simulink model "DC_gen_DC_PES"  (R2025a)
settings: Solver=VariableStepAuto  StartTime=0.0  StopTime=10.0  RelTol=1e-3
undefined symbols (not defined in the file): Grid_DCop_DC_PES
settings Model: Creator=atomas  LastModifiedBy=atomas

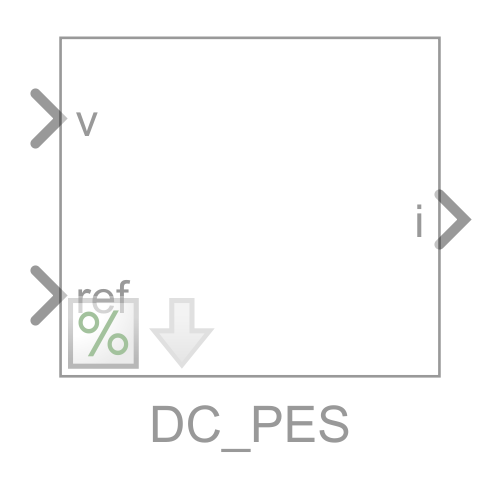
[thumbnail: Simulink's stored preview of the top-level diagram]
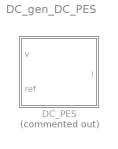
== system DC_gen_DC_PES ==
  DC_PES : Subsystem  Commented=on
      mask init:
      | mdlWks = get_param(bdroot,'ModelWorkspace'); % Get the model workspace
      | block_name = get_param(gcb,'Name');
      | try
      |     bvarname = get_param(get_param(get_param(...
      |         gcb, 'Parent'), 'Parent'), 'bvarname');
      |     DC = mdlWks.getVariable([bvarname 'DC']);
      |     block_buses = DC.([block_name 's_buses']);
      |     block_Pg = DC.([block_name 's_Pg']);
      |     block_toM = DC.([block_name 's_toM']);
      | catch ME % block in initialisation
      |     %errordlg(ME.message)
      |     try
      |         DC = mdlWks.getVariable('DC');
      |         block_buses = 1:length(DC.([block_name 's_buses']));
      |         block_Pg = DC.([block_name 's_Pg']);
      |         block_toM = eye(length(block_buses));
      |     catch ME
      |         %errordlg(ME.message)
      |     end
      | end

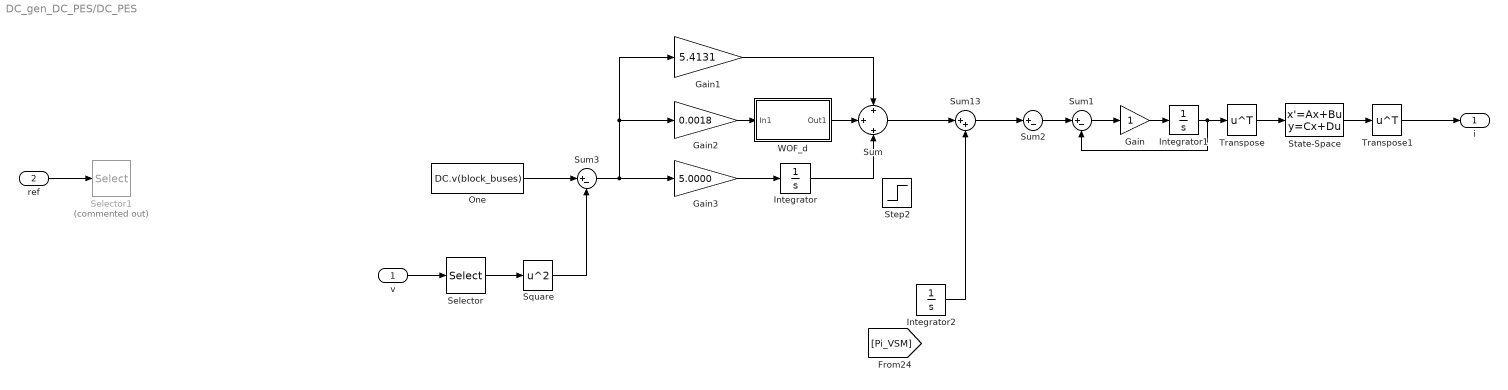
== system DC_gen_DC_PES/DC_PES ==
  v : Inport
  ref : Inport  Port=2
  Gain : Gain
  Gain1 : Gain  Gain=5.4131
  Gain2 : Gain  Gain=0.0018
  Gain3 : Gain  Gain=5.0000
  Integrator : Integrator  InitialCondition=Grid_DCop_DC_PES.op.States(1).x'
  Integrator1 : Integrator  InitialCondition=Grid_DCop_DC_PES.op.States(2).x'
  Integrator2 : Integrator  InitialCondition=Grid_DCop_DC_PES.op.States(3).x'
  One : Constant  Value=DC.v(block_buses)  VectorParams1D=off  OutDataTypeStr=Inherit: Inherit via back propagation
  Selector : Selector  InputPortWidth=DC.Nbuses  IndexOptions=Index vector (dialog)  Indices=block_buses  OutputSizes=1
  Selector1 : Selector  Commented=on  InputPortWidth=3  IndexOptions=Index vector (dialog)  Indices=[1 3]  OutputSizes=1
  Square : Math  Operator=square
  State-Space : StateSpace  A=[]  B=[]  C=[]  D=block_toM  InitialCondition=0  ParameterTunability=Optimized
  Step2 : Step  Time=0.1  After=0.1  SampleTime=0
  Sum : Sum  Inputs=+|+|+
  Sum1 : Sum  Inputs=|+-
  Sum13 : Sum  Inputs=|++
  Sum2 : Sum  Inputs=|+-
  Sum3 : Sum  Inputs=|+-
  Transpose : Math  Operator=transpose
  Transpose1 : Math  Operator=transpose
  WOF_d : Subsystem
  i : Outport
  wires:
  WOF_d/1(Out1) -> Sum/2
  Integrator/1 -> Sum/3
  Gain1/1 -> Sum/1
  Square/1 -> Sum3/2
  Gain3/1 -> Integrator/1
  Sum/1 -> Sum13/1
  Integrator2/1 -> Sum13/2
  Sum13/1 -> Sum2/1
  Gain2/1 -> WOF_d/1(In1)
  Sum2/1 -> Sum1/1
  Gain/1 -> Integrator1/1
  Integrator1/1 -> Transpose/1, Sum1/2
  Sum1/1 -> Gain/1
  One/1 -> Sum3/1
  Selector/1 -> Square/1
  v/1 -> Selector/1
  ref/1 -> Selector1/1
  Sum3/1 -> Gain3/1, Gain1/1, Gain2/1
  Transpose1/1 -> i/1
  Transpose/1 -> State-Space/1
  State-Space/1 -> Transpose1/1

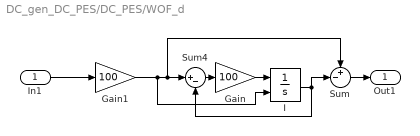
== system DC_gen_DC_PES/DC_PES/WOF_d ==
  In1 : Inport
  Gain : Gain  Gain=100
  Gain1 : Gain  Gain=100
  I : Integrator  InitialConditionSource=external  InitialCondition=Grid_DCop_DC_PES.op.States(4).x'
  Sum : Sum  Inputs=+-|
  Sum4 : Sum  Inputs=|+-
  Out1 : Outport
  wires:
  Gain1/1 -> Sum/1, Sum4/1, I/2
  Gain/1 -> I/1
  Sum4/1 -> Gain/1
  In1/1 -> Gain1/1
  I/1 -> Sum/2, Sum4/2
  Sum/1 -> Out1/1
